simulink model "PerturbedCartesianOrbitPropagator"  (R2023a)
settings: Solver=ode4  StartTime=0.0  StopTime=10.0  FixedStep=dt  MaxStep=max_step_size  RelTol=relative_tolerance
undefined symbols (not defined in the file or in its folder): plant
settings Model: Creator=ndelurgio  LastModifiedBy=ndelurgio

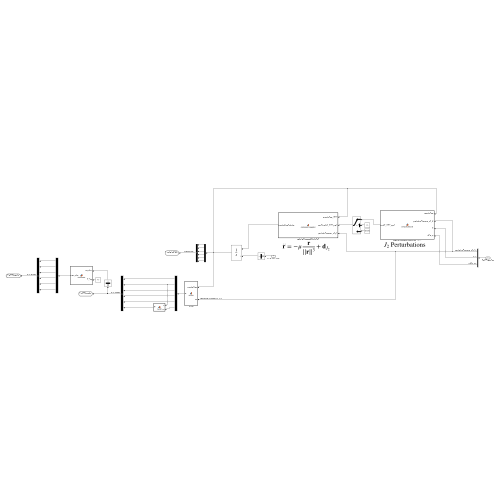
[thumbnail: Simulink's stored preview of the top-level diagram]
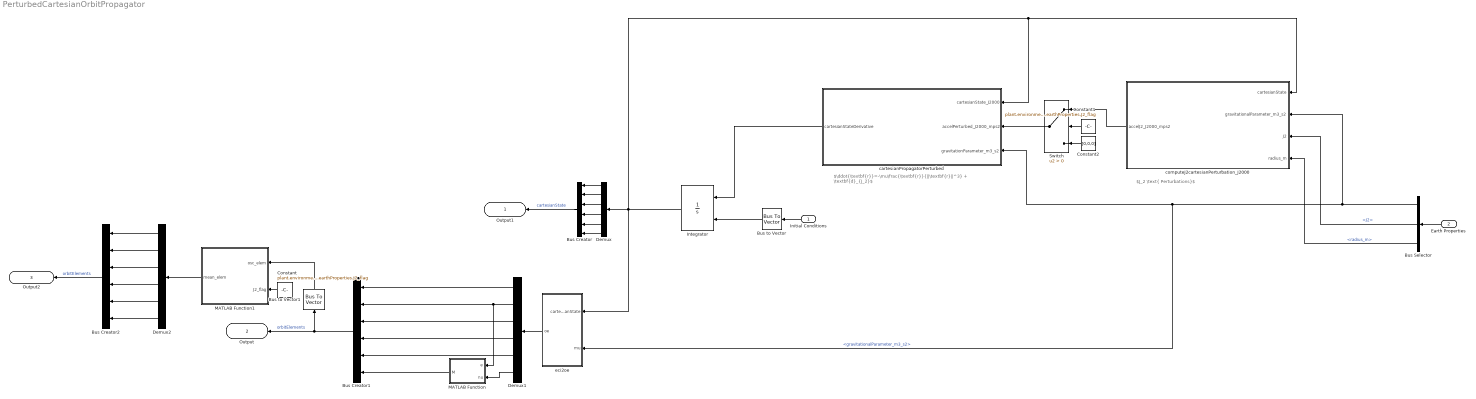
== system PerturbedCartesianOrbitPropagator ==
  note: $J_2 \text{ Perturbations}$
  note: $\ddot{\textbf{r}}=-\mu\frac{\textbf{r}}{||\textbf{r}||^3} + \textbf{d}_{J_2}$
  Initial Conditions : Inport  OutDataTypeStr=Bus: cartesianState
  Earth Properties : Inport  Port=2  OutDataTypeStr=Bus: earthProperties
  Bus Creator : BusCreator  Inputs=6  OutDataTypeStr=Bus: cartesianState  NonVirtualBus=on
      settings: InheritFromInputs=off
  Bus Creator1 : BusCreator  Inputs=6  OutDataTypeStr=Bus: osculatingOrbitElements
      settings: InheritFromInputs=off
  Bus Creator2 : BusCreator  Inputs=6  OutDataTypeStr=Bus: osculatingOrbitElements  NonVirtualBus=on
      settings: InheritFromInputs=off
  Bus Selector : BusSelector  OutputSignals=gravitationalParameter_m3_s2,J2,radius_m
  Bus to Vector : BusToVector
  Bus to Vector1 : BusToVector
  Constant : Constant  Value=plant.environment.earthProperties.J2_flag
  Constant1 : Constant  Value=plant.environment.earthProperties.J2_flag
  Constant2 : Constant  Value=[0,0,0]
  Demux : Demux  Outputs=6
  Demux1 : Demux  Outputs=6
  Demux2 : Demux  Outputs=6
  Integrator : Integrator  InitialConditionSource=external
  MATLAB Function : MATLAB Function  TreatAsAtomicUnit=on
  MATLAB Function1 : MATLAB Function  TreatAsAtomicUnit=on
  Switch : Switch  Criteria=u2 > Threshold  SaturateOnIntegerOverflow=off  InputSameDT=off
  cartesianPropagatorPerturbed : MATLAB Function  TreatAsAtomicUnit=on
  computeJ2cartesianPerturbation_J2000 : MATLAB Function  TreatAsAtomicUnit=on
  eci2oe : MATLAB Function  TreatAsAtomicUnit=on
  Output1 : Outport  OutDataTypeStr=Bus: cartesianState
  Output : Outport  Port=2  OutDataTypeStr=Bus: osculatingOrbitElements
  Output2 : Outport  Port=3  OutDataTypeStr=Bus: meanOrbitElements
  wires:
  computeJ2cartesianPerturbation_J2000/1(accelJ2_J2000_mps2) -> Switch/1
  Earth Properties/1 -> Bus Selector/1
  Bus Selector/2 -> computeJ2cartesianPerturbation_J2000/3(J2)  "<J2>"
  Bus Selector/3 -> computeJ2cartesianPerturbation_J2000/4(radius_m)  "<radius_m>"
  Demux/2 -> Bus Creator/2
  Bus Creator/1 -> Output1/1  "cartesianState"
  Demux/3 -> Bus Creator/3
  Demux/1 -> Bus Creator/1
  Demux/6 -> Bus Creator/6
  Demux/5 -> Bus Creator/5
  Demux/4 -> Bus Creator/4
  Bus to Vector/1 -> Integrator/2
  cartesianPropagatorPerturbed/1(cartesianStateDerivative) -> Integrator/1
  Initial Conditions/1 -> Bus to Vector/1
  eci2oe/1(oe) -> Demux1/1
  Bus Selector/1 -> eci2oe/2(mu), cartesianPropagatorPerturbed/3(gravitationParameter_m3_s2), computeJ2cartesianPerturbation_J2000/2(gravitationalParameter_m3_s2)  "<gravitationalParameter_m3_s2>"
  Integrator/1 -> eci2oe/1(cartesianState), computeJ2cartesianPerturbation_J2000/1(cartesianState), cartesianPropagatorPerturbed/1(cartesianState_J2000), Demux/1
  Demux1/6 -> MATLAB Function/2(nu)
  Demux1/4 -> Bus Creator1/4
  Demux1/5 -> Bus Creator1/5
  Bus Creator1/1 -> Bus to Vector1/1, Output/1  "orbitElements"
  Demux1/3 -> Bus Creator1/3
  Demux1/2 -> MATLAB Function/1(e), Bus Creator1/2
  Demux1/1 -> Bus Creator1/1
  MATLAB Function/1(M) -> Bus Creator1/6
  Bus to Vector1/1 -> MATLAB Function1/1(osc_elem)
  Constant/1 -> MATLAB Function1/2(J2_flag)
  MATLAB Function1/1(mean_elem) -> Demux2/1
  Demux2/4 -> Bus Creator2/4
  Demux2/3 -> Bus Creator2/3
  Demux2/5 -> Bus Creator2/5
  Demux2/2 -> Bus Creator2/2
  Demux2/1 -> Bus Creator2/1
  Demux2/6 -> Bus Creator2/6
  Bus Creator2/1 -> Output2/1  "orbitElements"
  Switch/1 -> cartesianPropagatorPerturbed/2(accelPerturbed_J2000_mps2)
  Constant1/1 -> Switch/2
  Constant2/1 -> Switch/3

== matlab function PerturbedCartesianOrbitPropagator/cartesianPropagatorPerturbed ==
  data: cartesianState_J2000 input; cartesianStateDerivative output; accelPerturbed_J2000_mps2 input; gravitationParameter_m3_s2 input
function cartesianStateDerivative = cartesianPropagator(cartesianState_J2000,accelPerturbed_J2000_mps2,gravitationParameter_m3_s2)

cartesianStateDerivative = cartesianPropagatorPerturbed(cartesianState_J2000,accelPerturbed_J2000_mps2,gravitationParameter_m3_s2);

end

== matlab function PerturbedCartesianOrbitPropagator/computeJ2cartesianPerturbation_J2000 ==
  data: cartesianState input; accelJ2_J2000_mps2 output; gravitationalParameter_m3_s2 input; J2 input; radius_m input
function accelJ2_J2000_mps2 = computeJ2accel(cartesianState,gravitationalParameter_m3_s2,J2,radius_m)

accelJ2_J2000_mps2 = computeJ2cartesianPerturbation_J2000(cartesianState,gravitationalParameter_m3_s2,J2,radius_m);

end

== matlab function PerturbedCartesianOrbitPropagator/eci2oe ==
  data: cartesianState input; oe output; mu input
function oe = eci2oe(cartesianState,mu)
[oe,~,~,~] = eci2oe( cartesianState , mu );
end

== matlab function PerturbedCartesianOrbitPropagator/MATLAB Function ==
  data: e input; M output; nu input
function M = nu2M(e,nu)
M = nu2M(nu,e);
end

== matlab function PerturbedCartesianOrbitPropagator/MATLAB Function1 ==
  data: osc_elem input; mean_elem output; J2_flag input
function mean_elem = osc2mean(osc_elem,J2_flag)
mean_elem = osc2mean(osc_elem,J2_flag);
end
